simulink model "Kalman_Filter_Simulink_Example"  (R2023b)
settings: Solver=VariableStepAuto  StartTime=0.0  StopTime=10  FixedStep=0.01  RelTol=1e-3
values from neighbouring files (symbols this model uses):
  A = [0 1; -g/l 0]    [Kalman_Filter_Simulink_Example_params.m]
  B = [0; 1/(m*l^2)]    [Kalman_Filter_Simulink_Example_params.m]
  C = [1 0]    [Kalman_Filter_Simulink_Example_params.m]
  D = 0    [Kalman_Filter_Simulink_Example_params.m]
  Q = 1e-3    (= 0.001)    [Kalman_Filter_Simulink_Example_params.m]
  R = 1e-4    (= 0.0001)    [Kalman_Filter_Simulink_Example_params.m]
  Ts = 0.01    [Kalman_Filter_Simulink_Example_params.m]
undefined symbols (not defined in the file or in its folder): Continuous, Time
libraries: simulink x2, ctrlSharedLib x1, Meldas_Library x1
settings Model: Creator=mulusoy  LastModifiedBy=leoni
settings SolverCC: AlgebraicLoopSolver=TrustRegion
settings DataIOCC: ReturnWorkspaceOutputs=off
settings OptimizationCC: DefaultParameterBehavior=Inlined  ReuseModelBlockBuffer=off  PassReuseOutputArgsAs=Individual arguments  EfficientTunableParamExpr=on
settings DebuggingCC: ParameterTunabilityLossMsg=error  UnconnectedInputMsg=warning  UnconnectedOutputMsg=warning  UnconnectedLineMsg=warning  ArithmeticOperatorsInVariantConditions=warning
settings ModelReferenceCC: EnableRefExpFcnMdlSchedulingChecks=on
settings SFSimCC: SimUseLocalCustomCode=off  MATLABDynamicMemAlloc=off  CustomCodeUndefinedFunction=UseInterfaceOnly
settings RTWCC: Description=Embedded Coder  SystemTargetFile=ert.tlc  TemplateMakefile=ert_default_tmf  GenerateReport=on  RTWUseLocalCustomCode=off  IncludeHyperlinkInReport=on  LaunchReport=on  GenerateTraceInfo=on  GenerateTraceReport=on  GenerateTraceReportSl=on  GenerateTraceReportSf=on  GenerateTraceReportEml=on  CheckMdlBeforeBuild=Warning
settings CodeAppCC: GenerateComments=off  IgnoreCustomStorageClasses=off  SimulinkBlockComments=off
settings ERTTargetCC: TargetLangStandard=C99 (ISO)  GenerateSampleERTMain=on  InlinedParameterPlacement=NonHierarchical  ERTCustomFileTemplate=example_file_process.tlc
settings SimscapeCC: SimscapeNormalizeSystem=off

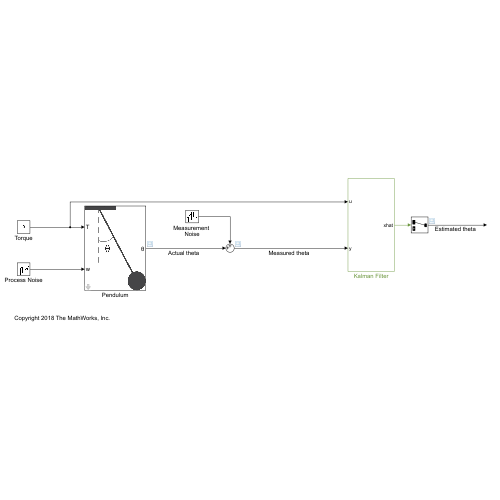
[thumbnail: Simulink's stored preview of the top-level diagram]
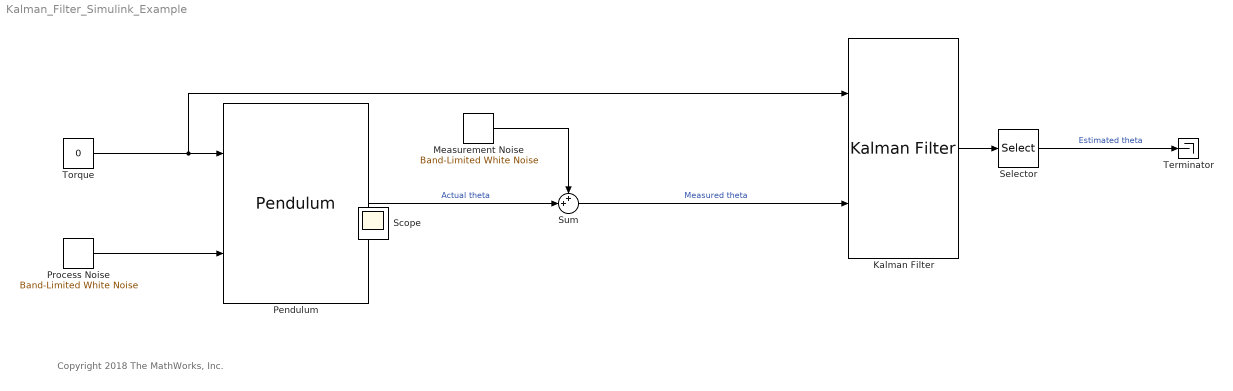
== system Kalman_Filter_Simulink_Example ==
  note: Copyright 2018 The MathWorks, Inc.
  Kalman Filter : ctrlSharedLib/Kalman Filter  TimeDomain=Continuous-Time  UseCurrentEstimator=on  ModelSource=Individual A, B, C, D matrices  ModelSourceVariable=ss(0.95,1,1,0,1)  A=A  B=B  C=C  D=D  NumberOfStates=1  NumberOfInputs=1  NumberOfOutputs=1  InitialEstimateSource=Dialog  X0=[pi/16 0]  P0=10  UseK=off  UseGH=off  NumberOfProcessNoiseInputs=1  G=1  TimeInvariantG=on  H=0  TimeInvariantH=on  Q=diag([0,Q])  TimeInvariantQ=on  R=R  TimeInvariantR=on  N=0  TimeInvariantN=on  AddInputPort=on  AddEnablePort=off  OutputEstimatedY=off  OutputP=off  Ts=0.01
  Measurement Noise : simulink/Sources/Band-Limited White Noise  Cov=R*Ts  Ts=Ts  seed=[12347]
  Pendulum : Meldas_Library/Pendulum  theta_0=pi/18  theta_dot_0=0
      link override Link/String: Density=2.7
  Process Noise : simulink/Sources/Band-Limited White Noise  Cov=Q*Ts  Ts=Ts  seed=[23341]
  Selector : Selector  InputPortWidth=2  IndexOptions=Index vector (dialog)  Indices=1  OutputSizes=1
  Sum : Sum  Inputs=++|
  Terminator : Terminator
  Torque : Constant  Value=0
  Scope : Scope
  wires:
  Pendulum/1 -> Sum/2  "Actual theta"
  Measurement Noise/1 -> Sum/1
  Sum/1 -> Kalman Filter/2  "Measured theta"
  Kalman Filter/1 -> Selector/1
  Selector/1 -> Terminator/1  "Estimated theta"
  Torque/1 -> Pendulum/1, Kalman Filter/1
  Process Noise/1 -> Pendulum/2
